simulink model "SATELLITE_ORBITE"  (R2013b)
settings: Solver=ode45  StartTime=0.0  StopTime=tfin  FixedStep=30  RelTol=1e-3
values from neighbouring files (symbols this model uses):
  f_perturb = [fr; ft]    [DYNORB.m]    (also in runSATELLITE_ORBITE.m = [0.0, -1.0e-05])
  GST_ini = 0.00    (= 0)    [TERRE.m]
  incl_ini = incl_ini_deg*deg2rad    [DYNORB.m]
  latsta = latsta_deg*deg2rad    [STATION.m]
  lonsta = lonsta_deg*deg2rad    [STATION.m]
  mu = 398601    [CONSTANTS.m]
  orb_ini = [r_ini,vr_ini,u_ini,wn_ini]    [DYNORB.m]
  possta_mod = re+altsta_m*m2km    [STATION.m]
  raan_ini = raan_ini_deg*deg2rad    [DYNORB.m]
  re = 6378.16    [CONSTANTS.m]
  RPY_O = [0, 1, 0 ... (first row only)    [CONSTANTS.m]
  Sun_incl_ini = Sun_incl_deg_ini*deg2rad    [SOLEIL.m]
  Sun_meanlong_ini = Sun_meanlong_deg_ini*deg2rad    [SOLEIL.m]
  Sun_mmot = 2*pi/(365.2422*24*3600)    (= 1.99106379729e-07)    [SOLEIL.m]
  we = 2*pi/persid    [TERRE.m]
settings Model: ExtModeAutoUpdateStatusClock=off  Creator=gaun2201  LastModifiedBy=Ouss
settings DataIOCC: SignalLoggingSaveFormat=ModelDataLogs  SignalLoggingName=sigsOut
settings OptimizationCC: ExpressionDepthLimit=2147483647  InitFltsAndDblsToZero=on
settings DebuggingCC: SaveWithParameterizedLinksMsg=none  SignalResolutionControl=TryResolveAllWithWarning  SolverPrmCheckMsg=none  MultiTaskDSMMsg=warning  MultiTaskCondExecSysMsg=none  FcnCallInpInsideContextMsg=UseLocalSettings  StateNameClashWarn=warning
settings HardwareCC: TargetUnknown=on
settings RTWCC: IncludeERTFirstTime=on
settings GRTTargetCC: TargetFcnLib=ansi_tfl_tmw.mat  CodeReplacementLibrary=None  ModelReferenceCompliant=off  ParMdlRefBuildCompliant=off  CompOptLevelCompliant=off  ConcurrentExecutionCompliant=off  CombineOutputUpdateFcns=off  MatFileLogging=off  CPPClassGenCompliant=on  GRTInterface=on

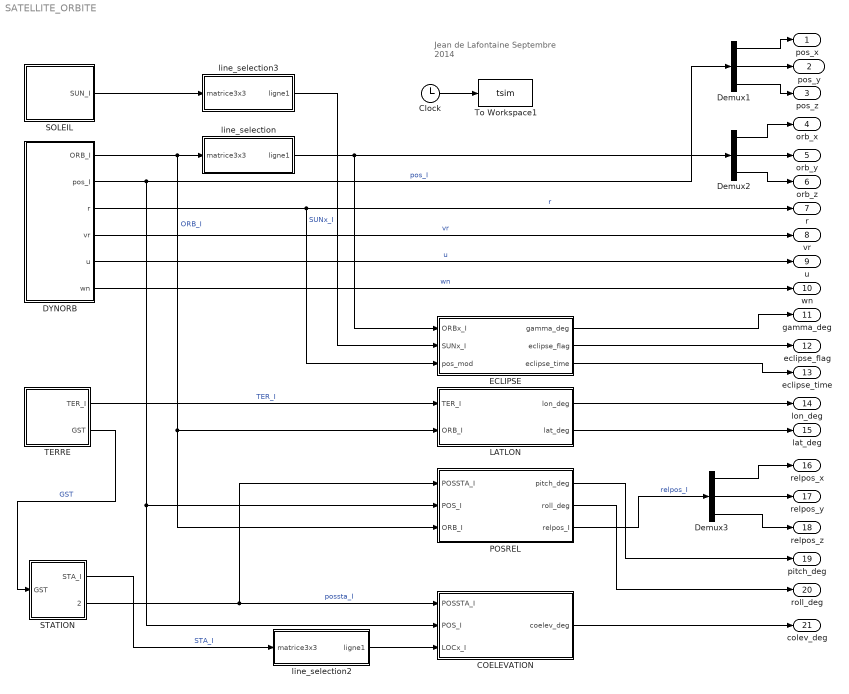
== system SATELLITE_ORBITE ==
  note: Jean de Lafontaine
      | Septembre 2014
  COELEVATION : Subsystem
  Clock : Clock
  DYNORB : Subsystem
  Demux1 : Demux  Outputs=3
  Demux2 : Demux  Outputs=3
  Demux3 : Demux  Outputs=3
  ECLIPSE : Subsystem
  LATLON : Subsystem
  POSREL : Subsystem
  SOLEIL : Subsystem
  STATION : Subsystem
  TERRE : Subsystem
  To Workspace1 : ToWorkspace  VariableName=tsim  SampleTime=-1
  line_selection : Subsystem
  line_selection2 : Subsystem
  line_selection3 : Subsystem
  pos_x : Outport
  pos_y : Outport  Port=2
  pos_z : Outport  Port=3
  orb_x : Outport  Port=4
  orb_y : Outport  Port=5
  orb_z : Outport  Port=6
  r : Outport  Port=7
  vr : Outport  Port=8
  u : Outport  Port=9
  wn : Outport  Port=10
  gamma_deg : Outport  Port=11
  eclipse_flag : Outport  Port=12
  eclipse_time : Outport  Port=13
  lon_deg : Outport  Port=14
  lat_deg : Outport  Port=15
  relpos_x : Outport  Port=16
  relpos_y : Outport  Port=17
  relpos_z : Outport  Port=18
  pitch_deg : Outport  Port=19
  roll_deg : Outport  Port=20
  colev_deg : Outport  Port=21
  wires:
  Clock/1 -> To Workspace1/1
  DYNORB/1(ORB_I) -> line_selection/1(matrice3x3), LATLON/2(ORB_I), POSREL/3(ORB_I)  "ORB_I"
  TERRE/1(TER_I) -> LATLON/1(TER_I)  "TER_I"
  line_selection2/1(ligne1) -> COELEVATION/3(LOCx_I)
  STATION/1(STA_I) -> line_selection2/1(matrice3x3)  "STA_I"
  TERRE/2(GST) -> STATION/1(GST)  "GST"
  line_selection/1(ligne1) -> ECLIPSE/1(ORBx_I), Demux2/1
  line_selection3/1(ligne1) -> ECLIPSE/2(SUNx_I)  "SUNx_I"
  SOLEIL/1(SUN_I) -> line_selection3/1(matrice3x3)
  ECLIPSE/1(gamma_deg) -> gamma_deg/1
  LATLON/1(lon_deg) -> lon_deg/1
  LATLON/2(lat_deg) -> lat_deg/1
  STATION/2(possta_I) -> POSREL/1(POSSTA_I), COELEVATION/1(POSSTA_I)  "possta_I"
  DYNORB/2(pos_I) -> POSREL/2(POS_I), COELEVATION/2(POS_I), Demux1/1  "pos_I"
  COELEVATION/1(coelev_deg) -> colev_deg/1
  POSREL/2(roll_deg) -> roll_deg/1
  POSREL/1(pitch_deg) -> pitch_deg/1
  Demux1/1 -> pos_x/1
  Demux1/3 -> pos_z/1
  Demux1/2 -> pos_y/1
  Demux2/1 -> orb_x/1
  Demux2/3 -> orb_z/1
  Demux2/2 -> orb_y/1
  POSREL/3(relpos_I) -> Demux3/1  "relpos_I"
  Demux3/1 -> relpos_x/1
  Demux3/2 -> relpos_y/1
  Demux3/3 -> relpos_z/1
  ECLIPSE/2(eclipse_flag) -> eclipse_flag/1
  DYNORB/3(r) -> r/1, ECLIPSE/3(pos_mod)  "r"
  DYNORB/4(vr) -> vr/1  "vr"
  DYNORB/5(u) -> u/1  "u"
  DYNORB/6(wn) -> wn/1  "wn"
  ECLIPSE/3(eclipse_time) -> eclipse_time/1

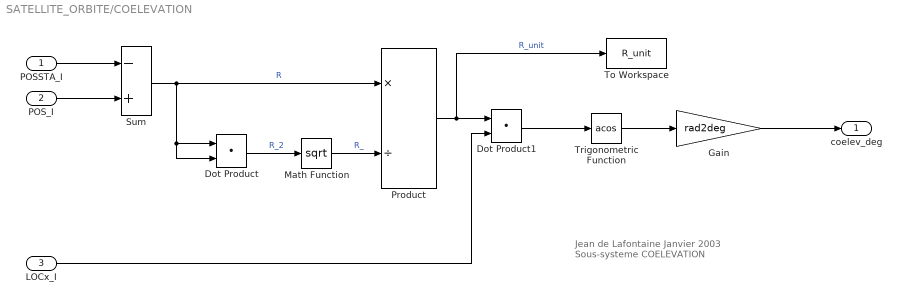
== system SATELLITE_ORBITE/COELEVATION ==
  note: Jean de Lafontaine
      | Janvier 2003
      |
      | Sous-systeme COELEVATION
  POSSTA_I : Inport
  POS_I : Inport  Port=2
  LOCx_I : Inport  Port=3
  Dot Product : DotProduct  InputSameDT=on  OutDataTypeStr=Inherit: Inherit via internal rule
  Dot Product1 : DotProduct  InputSameDT=on  OutDataTypeStr=Inherit: Inherit via internal rule
  Gain : Gain  Gain=rad2deg  SaturateOnIntegerOverflow=on  OutDataTypeStr=Inherit: Same as input  ParamDataTypeStr=Inherit: Same as input
  Math Function : Math  Operator=sqrt  SaturateOnIntegerOverflow=on
  Product : Product  Inputs=*/  SaturateOnIntegerOverflow=on  InputSameDT=on  OutDataTypeStr=Inherit: Same as first input
  Sum : Sum  Inputs=-+  SaturateOnIntegerOverflow=on  InputSameDT=on  OutDataTypeStr=Inherit: Same as first input
  To Workspace : ToWorkspace  VariableName=R_unit  SampleTime=-1
  Trigonometric Function : Trigonometry  Operator=acos
  coelev_deg : Outport
  wires:
  POS_I/1 -> Sum/2
  POSSTA_I/1 -> Sum/1
  Dot Product/1 -> Math Function/1  "R_2"
  Sum/1 -> Dot Product/2, Dot Product/1, Product/1  "R"
  Math Function/1 -> Product/2  "R_"
  Product/1 -> Dot Product1/1, To Workspace/1  "R_unit"
  Dot Product1/1 -> Trigonometric Function/1
  Trigonometric Function/1 -> Gain/1
  Gain/1 -> coelev_deg/1
  LOCx_I/1 -> Dot Product1/2

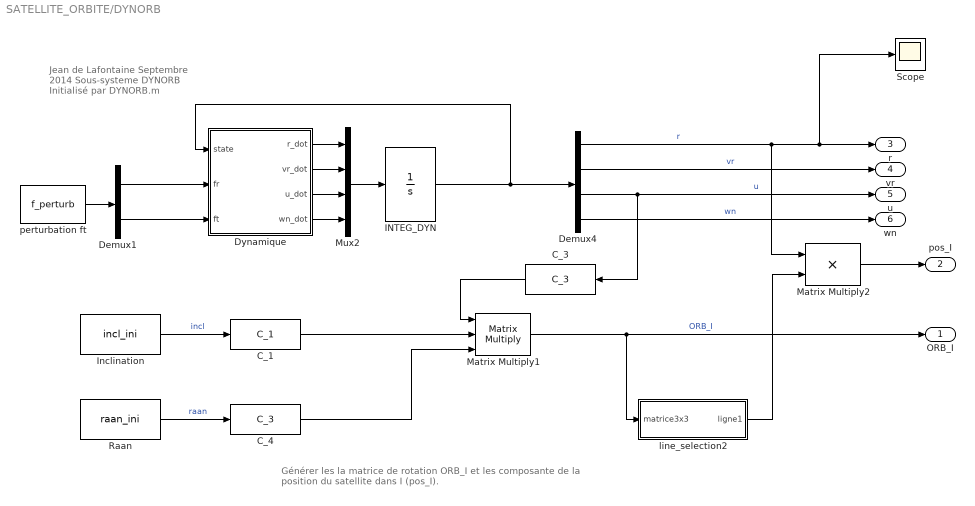
== system SATELLITE_ORBITE/DYNORB ==
  note: Jean de Lafontaine
      | Septembre 2014
      |
      | Sous-systeme DYNORB
      | Initialisé par DYNORB.m
  note: Générer les la matrice de rotation ORB_I et
      | les composante de la position du satellite dans I (pos_I).
  C_1 : MATLABFcn  MATLABFcn=C_1  Output1D=off
  C_3 : MATLABFcn  MATLABFcn=C_3  Output1D=off
  C_4 : MATLABFcn  MATLABFcn=C_3  Output1D=off
  Demux1 : Demux  Outputs=2
  Demux4 : Demux
  Dynamique : Subsystem
  INTEG_DYN : Integrator  InitialCondition=orb_ini
  Inclination : Constant  Value=incl_ini
  Matrix Multiply1 : Product  Inputs=3  Multiplication=Matrix(*)
  Matrix Multiply2 : Product
  Mux2 : Mux
  Raan : Constant  Value=raan_ini
  Scope : Scope
  line_selection2 : Subsystem
  perturbation ft : Constant  Value=f_perturb
  ORB_I : Outport
  pos_I : Outport  Port=2
  r : Outport  Port=3
  vr : Outport  Port=4
  u : Outport  Port=5
  wn : Outport  Port=6
  wires:
  Inclination/1 -> C_1/1  "incl"
  Matrix Multiply1/1 -> line_selection2/1(matrice3x3), ORB_I/1  "ORB_I"
  Raan/1 -> C_4/1  "raan"
  Matrix Multiply2/1 -> pos_I/1
  Dynamique/1(r_dot) -> Mux2/1
  Dynamique/2(vr_dot) -> Mux2/2
  Dynamique/3(u_dot) -> Mux2/3
  Dynamique/4(wn_dot) -> Mux2/4
  Mux2/1 -> INTEG_DYN/1
  INTEG_DYN/1 -> Dynamique/1(state), Demux4/1
  perturbation ft/1 -> Demux1/1
  Demux1/1 -> Dynamique/2(fr)
  Demux1/2 -> Dynamique/3(ft)
  Demux4/1 -> Matrix Multiply2/1, Scope/1, r/1  "r"
  Demux4/2 -> vr/1  "vr"
  Demux4/3 -> C_3/1, u/1  "u"
  Demux4/4 -> wn/1  "wn"
  C_4/1 -> Matrix Multiply1/3
  C_1/1 -> Matrix Multiply1/2
  C_3/1 -> Matrix Multiply1/1
  line_selection2/1(ligne1) -> Matrix Multiply2/2

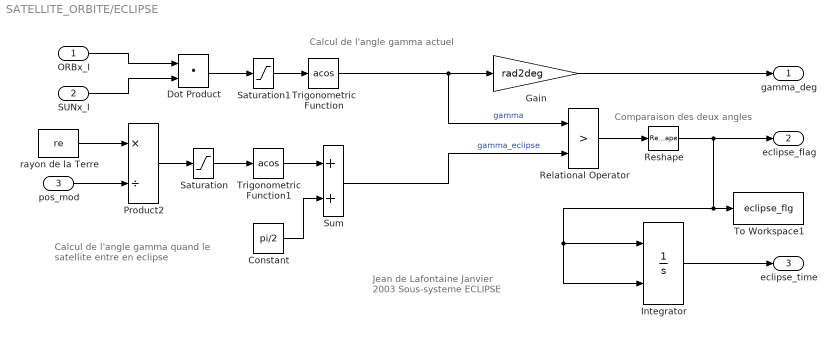
== system SATELLITE_ORBITE/ECLIPSE ==
  note: Jean de Lafontaine
      | Janvier 2003
      |
      | Sous-systeme ECLIPSE
  note: Calcul de l'angle gamma quand le
      | satellite entre en eclipse
  note: Calcul de l'angle gamma actuel
  note: Comparaison des deux angles
  ORBx_I : Inport
  SUNx_I : Inport  Port=2
  pos_mod : Inport  Port=3
  Constant : Constant  Value=pi/2
  Dot Product : DotProduct  InputSameDT=on  OutDataTypeStr=Inherit: Inherit via internal rule
  Gain : Gain  Gain=rad2deg  SaturateOnIntegerOverflow=on  OutDataTypeStr=Inherit: Same as input  ParamDataTypeStr=Inherit: Same as input
  Integrator : Integrator  ExternalReset=either
  Product2 : Product  Inputs=*/  SaturateOnIntegerOverflow=on  InputSameDT=on  OutDataTypeStr=Inherit: Same as first input
  Relational Operator : RelationalOperator  Operator=>  OutDataTypeStr='double'  InputSameDT=on
  Reshape : Reshape
  Saturation : Saturate  UpperLimit=1  LowerLimit=-1
  Saturation1 : Saturate  UpperLimit=1  LowerLimit=-1
  Sum : Sum  SaturateOnIntegerOverflow=on  InputSameDT=on  OutDataTypeStr=Inherit: Same as first input
  To Workspace1 : ToWorkspace  VariableName=eclipse_flg  SampleTime=-1
  Trigonometric Function : Trigonometry  Operator=acos
  Trigonometric Function1 : Trigonometry  Operator=acos
  rayon de la Terre : Constant  Value=re  VectorParams1D=off
  gamma_deg : Outport
  eclipse_flag : Outport  Port=2
  eclipse_time : Outport  Port=3
  wires:
  SUNx_I/1 -> Dot Product/2
  ORBx_I/1 -> Dot Product/1
  Dot Product/1 -> Saturation1/1
  Trigonometric Function/1 -> Gain/1, Relational Operator/1  "gamma"
  Gain/1 -> gamma_deg/1
  Sum/1 -> Relational Operator/2  "gamma_eclipse"
  Constant/1 -> Sum/2
  Trigonometric Function1/1 -> Sum/1
  Product2/1 -> Saturation/1
  pos_mod/1 -> Product2/2
  rayon de la Terre/1 -> Product2/1
  Saturation/1 -> Trigonometric Function1/1
  Saturation1/1 -> Trigonometric Function/1
  Integrator/1 -> eclipse_time/1
  Relational Operator/1 -> Reshape/1
  Reshape/1 -> eclipse_flag/1, To Workspace1/1, Integrator/2, Integrator/1

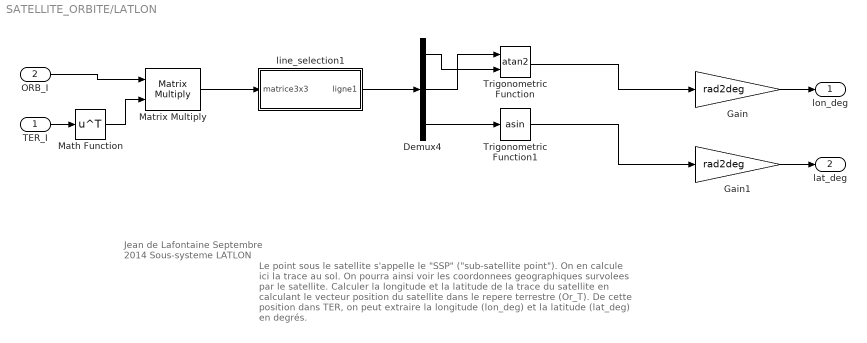
== system SATELLITE_ORBITE/LATLON ==
  note: Jean de Lafontaine
      | Septembre 2014
      |
      | Sous-systeme LATLON
  note: Le point sous le satellite s'appelle le "SSP" ("sub-satellite point").
      | On en calcule ici la trace au sol. On pourra ainsi voir les coordonnees
      | geographiques survolees par le satellite.
      |
      | Calculer la longitude et la latitude de la trace du satellite en calculant
      | le vecteur position du satellite dans le repere terrestre (Or_T). De cette
      | position dans TER, on peut extraire la longitude (lon_deg) et la
      | latitude (lat_deg) en degrés.
  TER_I : Inport
  ORB_I : Inport  Port=2
  Demux4 : Demux  Outputs=3
  Gain : Gain  Gain=rad2deg  SaturateOnIntegerOverflow=on  OutDataTypeStr=Inherit: Same as input  ParamDataTypeStr=Inherit: Same as input
  Gain1 : Gain  Gain=rad2deg  SaturateOnIntegerOverflow=on  OutDataTypeStr=Inherit: Same as input  ParamDataTypeStr=Inherit: Same as input
  Math Function : Math  Operator=transpose  SaturateOnIntegerOverflow=on
  Matrix Multiply : Product  Multiplication=Matrix(*)
  Trigonometric Function : Trigonometry  Operator=atan2
  Trigonometric Function1 : Trigonometry  Operator=asin
  line_selection1 : Subsystem
  lon_deg : Outport
  lat_deg : Outport  Port=2
  wires:
  Gain/1 -> lon_deg/1
  Gain1/1 -> lat_deg/1
  Matrix Multiply/1 -> line_selection1/1(matrice3x3)
  line_selection1/1(ligne1) -> Demux4/1
  Demux4/2 -> Trigonometric Function/1
  Demux4/1 -> Trigonometric Function/2
  Demux4/3 -> Trigonometric Function1/1
  Trigonometric Function/1 -> Gain/1
  Trigonometric Function1/1 -> Gain1/1
  TER_I/1 -> Math Function/1
  Math Function/1 -> Matrix Multiply/2
  ORB_I/1 -> Matrix Multiply/1

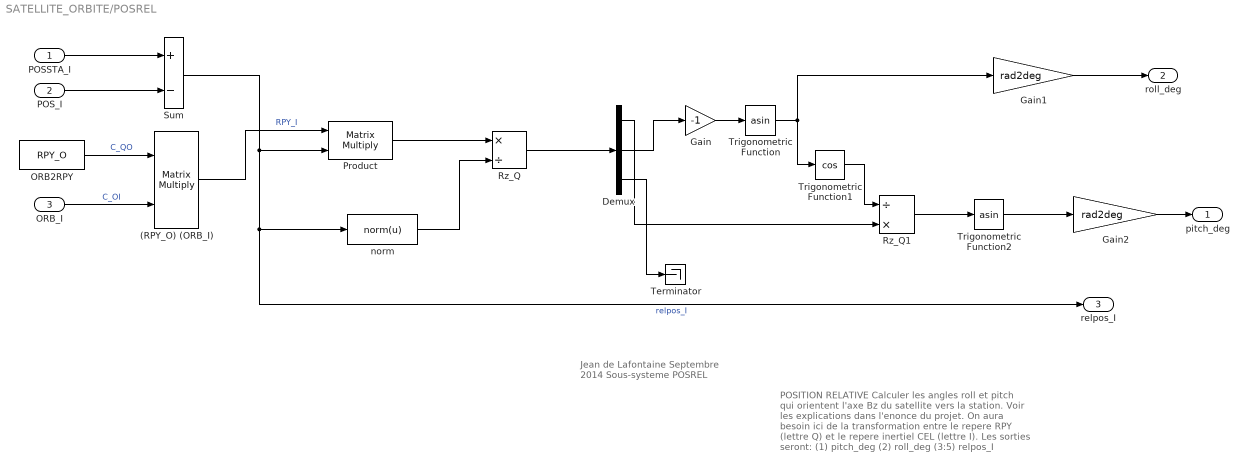
== system SATELLITE_ORBITE/POSREL ==
  note: Jean de Lafontaine
      | Septembre 2014
      |
      | Sous-systeme POSREL
  note: POSITION RELATIVE
      | Calculer les angles roll et pitch qui orientent
      | l'axe Bz du satellite vers la station. Voir les
      | explications dans l'enonce du projet. On aura
      | besoin ici de la transformation entre le repere
      | RPY (lettre Q) et le repere inertiel CEL (lettre I).
      | Les sorties seront:
      | (1)  pitch_deg
      | (2)  roll_deg
      | (3:5) relpos_I
  POSSTA_I : Inport
  POS_I : Inport  Port=2
  ORB_I : Inport  Port=3
  (RPY_O) (ORB_I) : Product  Multiplication=Matrix(*)  SaturateOnIntegerOverflow=on  InputSameDT=on  OutDataTypeStr=Inherit: Same as first input
  Demux : Demux  Outputs=3
  Gain : Gain  Gain=-1
  Gain1 : Gain  Gain=rad2deg  SaturateOnIntegerOverflow=on  OutDataTypeStr=Inherit: Same as input  ParamDataTypeStr=Inherit: Same as input
  Gain2 : Gain  Gain=rad2deg  SaturateOnIntegerOverflow=on  OutDataTypeStr=Inherit: Same as input  ParamDataTypeStr=Inherit: Same as input
  ORB2RPY : Constant  Value=RPY_O
  Product : Product  Multiplication=Matrix(*)
  Rz_Q : Product  Inputs=*/  SaturateOnIntegerOverflow=on  InputSameDT=on  OutDataTypeStr=Inherit: Same as first input
  Rz_Q1 : Product  Inputs=/*  SaturateOnIntegerOverflow=on  InputSameDT=on  OutDataTypeStr=Inherit: Same as first input
  Sum : Sum  Inputs=+-  SaturateOnIntegerOverflow=on  InputSameDT=on  OutDataTypeStr=Inherit: Same as first input
  Terminator : Terminator
  Trigonometric Function : Trigonometry  Operator=asin
  Trigonometric Function1 : Trigonometry  Operator=cos
  Trigonometric Function2 : Trigonometry  Operator=asin
  norm : MATLABFcn  MATLABFcn=norm(u)  Output1D=off
  pitch_deg : Outport
  roll_deg : Outport  Port=2
  relpos_I : Outport  Port=3
  wires:
  POS_I/1 -> Sum/2
  POSSTA_I/1 -> Sum/1
  ORB2RPY/1 -> (RPY_O) (ORB_I)/1  "C_QO"
  ORB_I/1 -> (RPY_O) (ORB_I)/2  "C_OI"
  Gain2/1 -> pitch_deg/1
  Gain1/1 -> roll_deg/1
  Sum/1 -> Product/2, norm/1, relpos_I/1  "relpos_I"
  Trigonometric Function/1 -> Trigonometric Function1/1, Gain1/1
  (RPY_O) (ORB_I)/1 -> Product/1  "RPY_I"
  Product/1 -> Rz_Q/1
  norm/1 -> Rz_Q/2
  Rz_Q/1 -> Demux/1
  Gain/1 -> Trigonometric Function/1
  Demux/3 -> Terminator/1
  Trigonometric Function1/1 -> Rz_Q1/1
  Rz_Q1/1 -> Trigonometric Function2/1
  Demux/2 -> Gain/1
  Demux/1 -> Rz_Q1/2
  Trigonometric Function2/1 -> Gain2/1

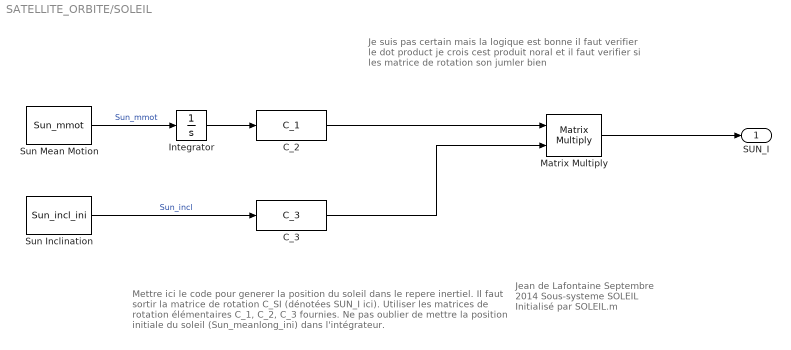
== system SATELLITE_ORBITE/SOLEIL ==
  note: Je suis pas certain mais la logique est bonne
      | il faut verifier le dot product je crois cest produit noral
      | et il faut verifier si les matrice de rotation son jumler bien
  note: Jean de Lafontaine
      | Septembre 2014
      |
      | Sous-systeme SOLEIL
      | Initialisé par SOLEIL.m
  note: Mettre ici le code pour generer la position du soleil dans le repere
      | inertiel. Il faut sortir la matrice de rotation C_SI (dénotées SUN_I ici).
      | Utiliser les matrices de rotation élémentaires C_1, C_2, C_3 fournies.
      | Ne pas oublier de mettre la position initiale du soleil (Sun_meanlong_ini)
      | dans l'intégrateur.
  C_2 : MATLABFcn  MATLABFcn=C_1  Output1D=off
  C_3 : MATLABFcn  MATLABFcn=C_3  Output1D=off
  Integrator : Integrator  InitialCondition=Sun_meanlong_ini
  Matrix Multiply : Product  Multiplication=Matrix(*)
  Sun Inclination : Constant  Value=Sun_incl_ini
  Sun Mean Motion : Constant  Value=Sun_mmot
  SUN_I : Outport
  wires:
  Sun Mean Motion/1 -> Integrator/1  "Sun_mmot"
  Sun Inclination/1 -> C_3/1  "Sun_incl"
  Matrix Multiply/1 -> SUN_I/1
  Integrator/1 -> C_2/1
  C_2/1 -> Matrix Multiply/1
  C_3/1 -> Matrix Multiply/2

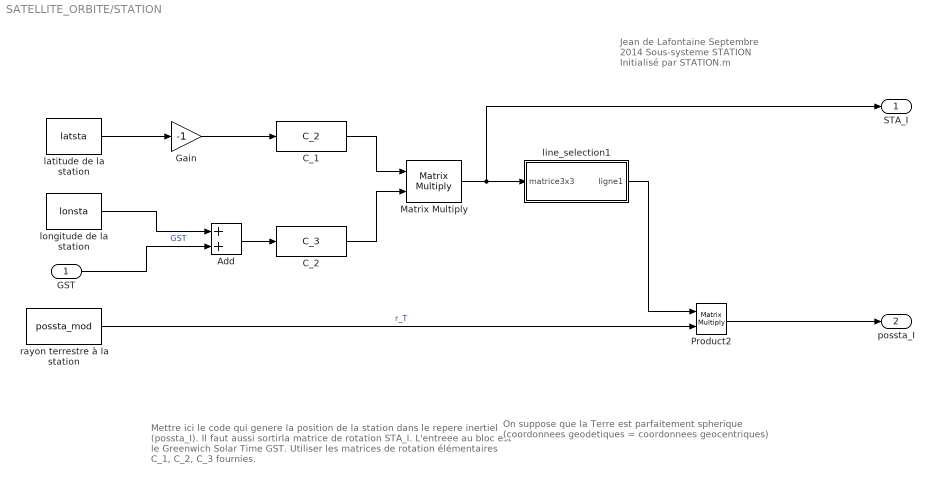
== system SATELLITE_ORBITE/STATION ==
  note: Jean de Lafontaine
      | Septembre 2014
      |
      | Sous-systeme STATION
      | Initialisé par STATION.m
  note: Mettre ici le code qui genere la position de la station dans le repere
      | inertiel (possta_I). Il faut aussi sortirla matrice de rotation STA_I.
      | L'entreee au bloc est le Greenwich Solar Time GST.
      | Utiliser les matrices de rotation élémentaires C_1, C_2, C_3 fournies.
  note: On suppose que la Terre est parfaitement spherique
      | (coordonnees geodetiques = coordonnees geocentriques)
  GST : Inport
  Add : Sum
  C_1 : MATLABFcn  MATLABFcn=C_2  Output1D=off
  C_2 : MATLABFcn  MATLABFcn=C_3  Output1D=off
  Gain : Gain  Gain=-1
  Matrix Multiply : Product  Multiplication=Matrix(*)
  Product2 : Product  Multiplication=Matrix(*)
  latitude de la station : Constant  Value=latsta  VectorParams1D=off
  line_selection1 : Subsystem
  longitude de la station : Constant  Value=lonsta  VectorParams1D=off
  rayon terrestre à la station : Constant  Value=possta_mod  VectorParams1D=off
  STA_I : Outport
  possta_I : Outport  Port=2
  wires:
  latitude de la station/1 -> Gain/1
  longitude de la station/1 -> Add/1
  GST/1 -> Add/2  "GST"
  Product2/1 -> possta_I/1
  Matrix Multiply/1 -> STA_I/1, line_selection1/1(matrice3x3)
  rayon terrestre à la station/1 -> Product2/2  "r_T"
  Add/1 -> C_2/1
  Gain/1 -> C_1/1
  C_1/1 -> Matrix Multiply/1
  C_2/1 -> Matrix Multiply/2
  line_selection1/1(ligne1) -> Product2/1

== system SATELLITE_ORBITE/TERRE ==
  note: Jean de Lafontaine
      | Janvier 2003
      |
      | Sous-systeme TERRE
      | Initialisé par TERRE.m
  note: TER_I est la matrice de rotation C_TI
      | GST est aussi utilisé dans le module 'STATION'.
  C_3 : MATLABFcn  MATLABFcn=C_3  Output1D=off
  GST_ini : Integrator  InitialCondition=GST_ini
  vitesse de rotation de la terre : Constant  Value=we
  TER_I : Outport
  GST : Outport  Port=2
  wires:
  vitesse de rotation de la terre/1 -> GST_ini/1
  GST_ini/1 -> C_3/1, GST/1  "GST"
  C_3/1 -> TER_I/1

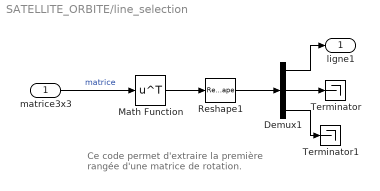
== system SATELLITE_ORBITE/line_selection ==
  note: Ce code permet d'extraire la première
      | rangée d'une matrice de rotation.
  matrice3x3 : Inport
  Demux1 : Demux  Outputs=[3,3,3]
  Math Function : Math  Operator=transpose  SaturateOnIntegerOverflow=on
  Reshape1 : Reshape
  Terminator : Terminator
  Terminator1 : Terminator
  ligne1 : Outport
  wires:
  matrice3x3/1 -> Math Function/1  "matrice"
  Math Function/1 -> Reshape1/1
  Demux1/1 -> ligne1/1
  Demux1/2 -> Terminator/1
  Demux1/3 -> Terminator1/1
  Reshape1/1 -> Demux1/1

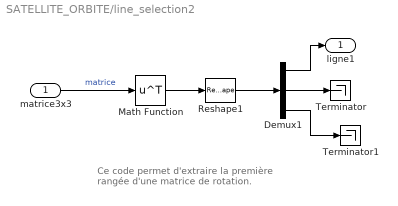
== system SATELLITE_ORBITE/line_selection2 ==
  note: Ce code permet d'extraire la première
      | rangée d'une matrice de rotation.
  matrice3x3 : Inport
  Demux1 : Demux  Outputs=[3,3,3]
  Math Function : Math  Operator=transpose  SaturateOnIntegerOverflow=on
  Reshape1 : Reshape
  Terminator : Terminator
  Terminator1 : Terminator
  ligne1 : Outport
  wires:
  matrice3x3/1 -> Math Function/1  "matrice"
  Math Function/1 -> Reshape1/1
  Demux1/1 -> ligne1/1
  Demux1/2 -> Terminator/1
  Demux1/3 -> Terminator1/1
  Reshape1/1 -> Demux1/1

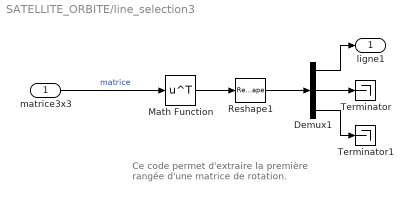
== system SATELLITE_ORBITE/line_selection3 ==
  note: Ce code permet d'extraire la première
      | rangée d'une matrice de rotation.
  matrice3x3 : Inport
  Demux1 : Demux  Outputs=[3,3,3]
  Math Function : Math  Operator=transpose  SaturateOnIntegerOverflow=on
  Reshape1 : Reshape
  Terminator : Terminator
  Terminator1 : Terminator
  ligne1 : Outport
  wires:
  matrice3x3/1 -> Math Function/1  "matrice"
  Math Function/1 -> Reshape1/1
  Demux1/1 -> ligne1/1
  Demux1/2 -> Terminator/1
  Demux1/3 -> Terminator1/1
  Reshape1/1 -> Demux1/1

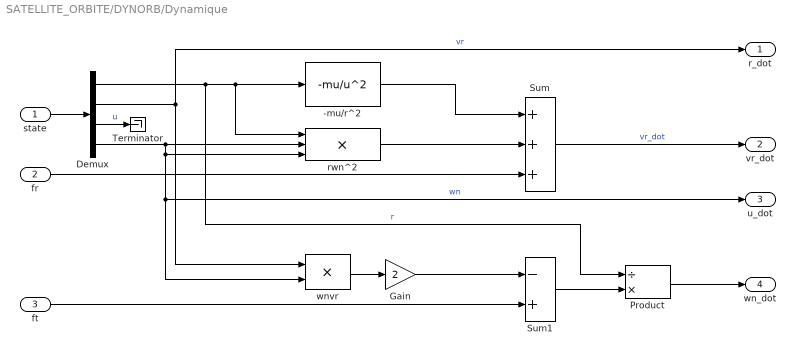
== system SATELLITE_ORBITE/DYNORB/Dynamique ==
  state : Inport
  fr : Inport  Port=2
  ft : Inport  Port=3
  -mu/r^2 : Fcn  Expr=-mu/u^2
  Demux : Demux
  Gain : Gain  Gain=2  SaturateOnIntegerOverflow=on  OutDataTypeStr=Inherit: Same as input  ParamDataTypeStr=Inherit: Same as input
  Product : Product  Inputs=/*  SaturateOnIntegerOverflow=on  InputSameDT=on  OutDataTypeStr=Inherit: Same as first input
  Sum : Sum  Inputs=+++  SaturateOnIntegerOverflow=on  InputSameDT=on  OutDataTypeStr=Inherit: Same as first input
  Sum1 : Sum  Inputs=-+  SaturateOnIntegerOverflow=on  InputSameDT=on  OutDataTypeStr=Inherit: Same as first input
  Terminator : Terminator
  rwn^2 : Product  Inputs=3  SaturateOnIntegerOverflow=on  InputSameDT=on  OutDataTypeStr=Inherit: Same as first input
  wnvr : Product  SaturateOnIntegerOverflow=on  InputSameDT=on  OutDataTypeStr=Inherit: Same as first input
  r_dot : Outport
  vr_dot : Outport  Port=2
  u_dot : Outport  Port=3
  wn_dot : Outport  Port=4
  wires:
  state/1 -> Demux/1
  Demux/4 -> wnvr/2, u_dot/1, rwn^2/3, rwn^2/2  "wn"
  Demux/1 -> Product/1, -mu/r^2/1, rwn^2/1  "r"
  Demux/2 -> wnvr/1, r_dot/1  "vr"
  -mu/r^2/1 -> Sum/1
  rwn^2/1 -> Sum/2
  fr/1 -> Sum/3
  Sum/1 -> vr_dot/1  "vr_dot"
  wnvr/1 -> Gain/1
  Gain/1 -> Sum1/1
  ft/1 -> Sum1/2
  Sum1/1 -> Product/2
  Product/1 -> wn_dot/1
  Demux/3 -> Terminator/1  "u"

== system SATELLITE_ORBITE/DYNORB/line_selection2 ==
  note: Ce code permet d'extraire la première
      | rangée d'une matrice de rotation.
  matrice3x3 : Inport
  Demux1 : Demux  Outputs=[3,3,3]
  Math Function : Math  Operator=transpose  SaturateOnIntegerOverflow=on
  Reshape1 : Reshape
  Terminator : Terminator
  Terminator1 : Terminator
  ligne1 : Outport
  wires:
  matrice3x3/1 -> Math Function/1  "matrice"
  Math Function/1 -> Reshape1/1
  Demux1/1 -> ligne1/1
  Demux1/2 -> Terminator/1
  Demux1/3 -> Terminator1/1
  Reshape1/1 -> Demux1/1

== system SATELLITE_ORBITE/LATLON/line_selection1 ==
  note: Ce code permet d'extraire la première
      | rangée d'une matrice de rotation.
  matrice3x3 : Inport
  Demux1 : Demux  Outputs=[3,3,3]
  Math Function : Math  Operator=transpose  SaturateOnIntegerOverflow=on
  Reshape1 : Reshape
  Terminator : Terminator
  Terminator1 : Terminator
  ligne1 : Outport
  wires:
  matrice3x3/1 -> Math Function/1  "matrice"
  Math Function/1 -> Reshape1/1
  Demux1/1 -> ligne1/1
  Demux1/2 -> Terminator/1
  Demux1/3 -> Terminator1/1
  Reshape1/1 -> Demux1/1

== system SATELLITE_ORBITE/STATION/line_selection1 ==
  note: Ce code permet d'extraire la première
      | rangée d'une matrice de rotation.
  matrice3x3 : Inport
  Demux1 : Demux  Outputs=[3,3,3]
  Math Function : Math  Operator=transpose  SaturateOnIntegerOverflow=on
  Reshape1 : Reshape
  Terminator : Terminator
  Terminator1 : Terminator
  ligne1 : Outport
  wires:
  matrice3x3/1 -> Math Function/1  "matrice"
  Math Function/1 -> Reshape1/1
  Demux1/1 -> ligne1/1
  Demux1/2 -> Terminator/1
  Demux1/3 -> Terminator1/1
  Reshape1/1 -> Demux1/1
